simulink library "ExtractCovDiag"  (R2018b)
settings: Solver=VariableStepAuto  StartTime=0.0  StopTime=10.0  RelTol=1e-3
settings Model: Creator=BI28030  LastModifiedBy=BI28030

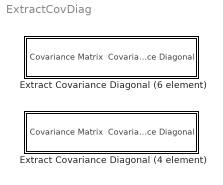
== system ExtractCovDiag ==
  Extract Covariance Diagonal (4 element) : Subsystem
  Extract Covariance Diagonal (6 element) : Subsystem

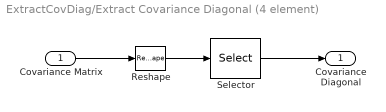
== system ExtractCovDiag/Extract Covariance Diagonal (4 element) ==
  Covariance Matrix : Inport
  Reshape : Reshape
  Selector : Selector  InputPortWidth=16  IndexOptions=Index vector (dialog)  Indices=[1,6,11,16]  OutputSizes=1
  Covariance Diagonal : Outport
  wires:
  Selector/1 -> Covariance Diagonal/1
  Covariance Matrix/1 -> Reshape/1
  Reshape/1 -> Selector/1

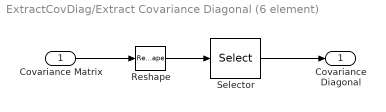
== system ExtractCovDiag/Extract Covariance Diagonal (6 element) ==
  Covariance Matrix : Inport
  Reshape : Reshape
  Selector : Selector  InputPortWidth=36  IndexOptions=Index vector (dialog)  Indices=[1 8 15 22 29 36]  OutputSizes=1
  Covariance Diagonal : Outport
  wires:
  Selector/1 -> Covariance Diagonal/1
  Covariance Matrix/1 -> Reshape/1
  Reshape/1 -> Selector/1
